simulink model "Model"  (R2024a)
settings: Solver=VariableStepAuto  StartTime=0.0  StopTime=30  RelTol=1e-3
values from neighbouring files (symbols this model uses):
  u_trim = ZStar(10:13)    [Trim_UAV.m]    (also in main.m)
  x_trim = ZStar(1:9)    [Trim_UAV.m]    (also in main.m)
undefined symbols (not defined in the file or in its folder): P, UAV_Morphing_MODEL
libraries: sharedtransform x1
settings Model: Creator=Mustafa Taha  LastModifiedBy=Mustafa Taha

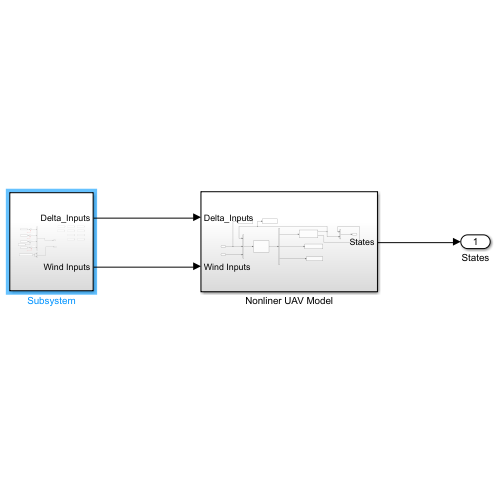
[thumbnail: Simulink's stored preview of the top-level diagram]
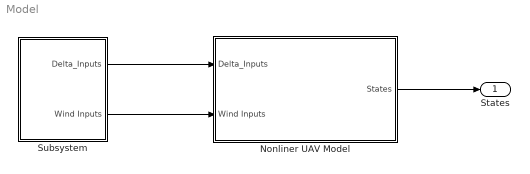
== system Model ==
  Nonliner UAV Model : Subsystem
  Subsystem : Subsystem
  States : Outport
  wires:
  Nonliner UAV Model/1(States) -> States/1
  Subsystem/1(Delta_Inputs) -> Nonliner UAV Model/1(Delta_Inputs)
  Subsystem/2(Wind Inputs) -> Nonliner UAV Model/2(Wind Inputs)

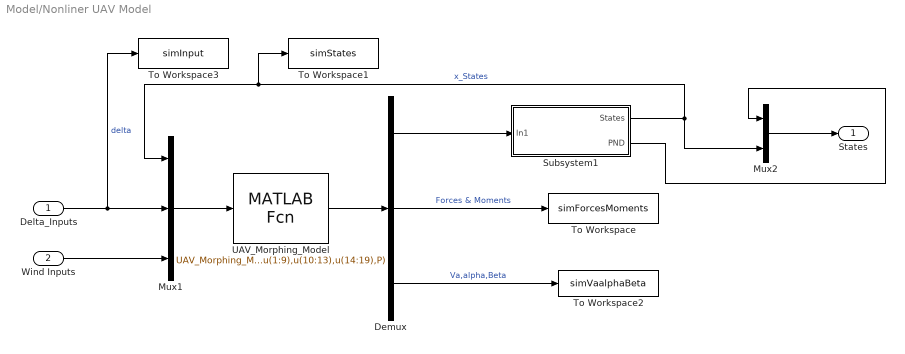
== system Model/Nonliner UAV Model ==
  Delta_Inputs : Inport
  Wind Inputs : Inport  Port=2
  Demux : Demux  Outputs=[9;6;6]
  Mux1 : Mux  Inputs=3
  Mux2 : Mux  Inputs=2
  Subsystem1 : Subsystem
  To Workspace : ToWorkspace  VariableName=simForcesMoments  SaveFormat=Timeseries  SampleTime=-1
  To Workspace1 : ToWorkspace  VariableName=simStates  SaveFormat=Timeseries  SampleTime=-1
  To Workspace2 : ToWorkspace  VariableName=simVaalphaBeta  SaveFormat=Timeseries  SampleTime=-1
  To Workspace3 : ToWorkspace  VariableName=simInput  SaveFormat=Timeseries  SampleTime=-1
  UAV_Morphing_Model : MATLABFcn  MATLABFcn=UAV_Morphing_MODEL(u(1:9),u(10:13),u(14:19),P)  OutputDimensions=21
  States : Outport
  wires:
  Mux1/1 -> UAV_Morphing_Model/1
  Demux/1 -> Subsystem1/1(In1)
  Subsystem1/1(States) -> Mux2/2, To Workspace1/1, Mux1/1  "x_States"
  Wind Inputs/1 -> Mux1/3
  Subsystem1/2(PND) -> Mux2/1
  UAV_Morphing_Model/1 -> Demux/1
  Demux/2 -> To Workspace/1  "Forces & Moments"
  Demux/3 -> To Workspace2/1  "Va,alpha,Beta"
  Mux2/1 -> States/1
  Delta_Inputs/1 -> To Workspace3/1, Mux1/2  "delta"

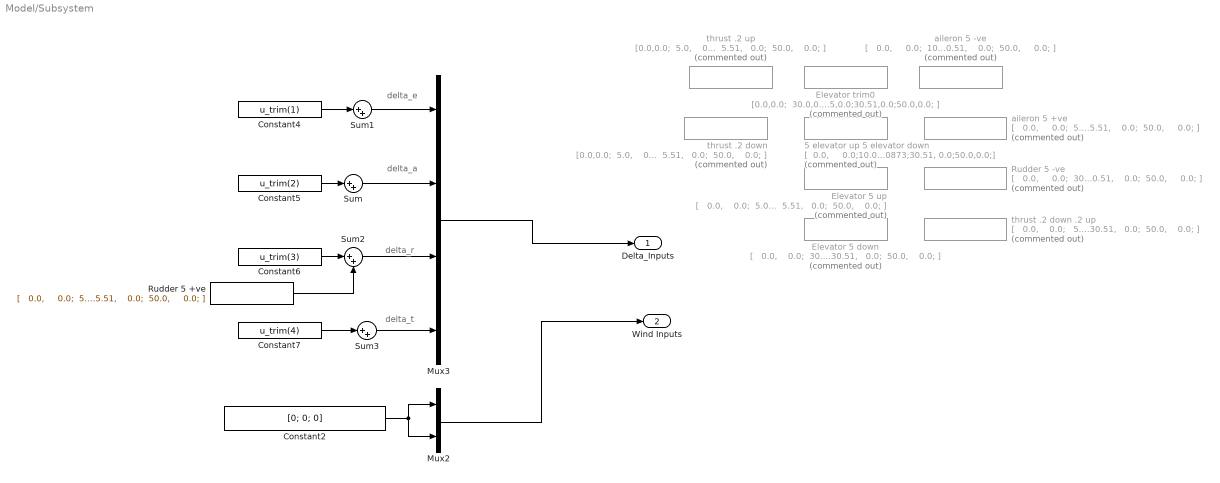
== system Model/Subsystem ==
  note: delta_a
  note: delta_t
  note: delta_e
  note: delta_r
  5 elevator up 5 elevator down : FromWorkspace  Commented=on  VariableName="[  0.0,     0.0;10.0, 0.0;10.01,  -0.0873;10.5,   -0.0873; 10.51,   0.0;30.0,    0.0;30.01,   0.0873;30.5,    0.0873;30.51, 0.0;50.0,0.0;]"
  Constant2 : Constant  Value=[0; 0; 0]
  Constant4 : Constant  Value=u_trim(1)
  Constant5 : Constant  Value=u_trim(2)
  Constant6 : Constant  Value=u_trim(3)
  Constant7 : Constant  Value=u_trim(4)
  Elevator 5 down : FromWorkspace  Commented=on  VariableName=|
      | [
      |   0.0,    0.0;
      |  30.0,    0.0;
      |  30.01,   0.0873;
      |  30.5,    0.0873;
      |  30.51,   0.0;
      |  50.0,    0.0;
      | ]
  Elevator 5 up : FromWorkspace  Commented=on  VariableName=|
      | [
      |   0.0,    0.0;
      |  5.0,    0.0;
      |  5.01,   -0.0873;
      |  5.5,   -0.0873;
      |  5.51,   0.0;
      |  50.0,    0.0;
      | ]
  Elevator trim0 : FromWorkspace  Commented=on  VariableName=|
      | [0.0,0.0;
      |  30.0,0.0;30.01,0.0;30.5,0.0;30.51,0.0;50.0,0.0;
      | ]
  Mux2 : Mux  Inputs=2
  Mux3 : Mux
  Rudder 5 +ve : FromWorkspace  VariableName=|
      | [
      |   0.0,     0.0;
      |  5.0,     0.0;
      |  5.01,   0.0873;
      |  5.5,    0.0873;
      |  5.51,    0.0;
      |  50.0,     0.0;
      | ]
  Rudder 5 -ve : FromWorkspace  Commented=on  VariableName=|
      | [
      |   0.0,     0.0;
      |  30.0,     0.0;
      |  30.01,   -0.0873;
      |  30.5,    -0.0873;
      |  30.51,    0.0;
      |  50.0,     0.0;
      | ]
  Sum{,1..3} (4 alike) : Sum  Inputs=|++
  aileron 5 +ve : FromWorkspace  Commented=on  VariableName=|
      | [
      |   0.0,     0.0;
      |  5.0,     0.0;
      |  5.01,    0.0873;
      |  5.5,     0.0873;
      |  5.51,    0.0;
      |  50.0,     0.0;
      | ]
  aileron 5 -ve : FromWorkspace  Commented=on  VariableName=|
      | [
      |   0.0,     0.0;
      |  10.0,     0.0;
      |  10.01,   -0.0436;
      |  10.5,    -0.0436;
      |  10.51,    0.0;
      |  50.0,     0.0;
      | ]
  thrust .2 down : FromWorkspace  Commented=on  VariableName=|
      | [0.0,0.0;
      |  5.0,    0.0;
      |  5.01,  -0.2;
      |  5.5,   -0.2;
      |  5.51,   0.0;
      |  50.0,    0.0;
      | ]
  thrust .2 down .2 up : FromWorkspace  Commented=on  VariableName=|
      | [
      |   0.0,    0.0;
      |   5.0,    0.0;
      |   5.01,  0.2;
      |   5.5,   0.2;
      |   5.51,   0.0;
      |  30.0,    0.0;
      |  30.01,   -0.2;
      |  30.5,    -0.2;
      |  30.51,   0.0;
      |  50.0,    0.0;
      | ]
  thrust .2 up : FromWorkspace  Commented=on  VariableName=|
      | [0.0,0.0;
      |  5.0,    0.0;
      |  5.01,  0.2;
      |  5.5,   0.2;
      |  5.51,   0.0;
      |  50.0,    0.0;
      | ]
  Delta_Inputs : Outport
  Wind Inputs : Outport  Port=2
  wires:
  Sum2/1 -> Mux3/3
  Constant2/1 -> Mux2/1, Mux2/2
  Constant6/1 -> Sum2/1
  Sum1/1 -> Mux3/1
  Mux2/1 -> Wind Inputs/1
  Constant7/1 -> Sum3/1
  Constant4/1 -> Sum1/1
  Sum/1 -> Mux3/2
  Constant5/1 -> Sum/1
  Mux3/1 -> Delta_Inputs/1
  Sum3/1 -> Mux3/4
  ? -> Sum/2
  ? -> Sum1/2
  ? -> Sum3/2
  Rudder 5 +ve/1 -> Sum2/2

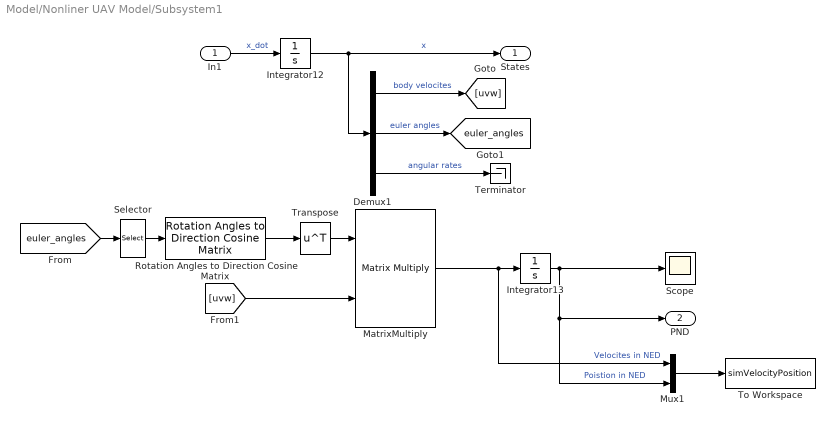
== system Model/Nonliner UAV Model/Subsystem1 ==
  In1 : Inport
  Demux1 : Demux  Outputs=[3,3,3]
  Integrator12 : Integrator  InitialCondition=x_trim
  Integrator13 : Integrator  InitialCondition=[0;0;-100]
  MatrixMultiply : Product  Multiplication=Matrix(*)
  Mux1 : Mux  Inputs=2
  Rotation Angles to Direction Cosine Matrix : sharedtransform/Rotation Angles to Direction Cosine Matrix  rotationOrder=ZYX  aMode=aMode
  Scope : Scope
  Selector : Selector  InputPortWidth=3  IndexOptions=Index vector (dialog)  Indices=[3 2 1]  OutputSizes=1
  Terminator : Terminator
  To Workspace : ToWorkspace  VariableName=simVelocityPosition  SaveFormat=Timeseries  SampleTime=-1
  Transpose : Math  Operator=transpose
  States : Outport
  PND : Outport  Port=2
  tag scope: euler_angles=global
  wires:
  In1/1 -> Integrator12/1  "x_dot"
  Integrator12/1 -> Demux1/1, States/1  "x"
  Integrator13/1 -> PND/1, Mux1/2, Scope/1  "Poistion in NED"
  [euler_angles] -> Selector/1
  Selector/1 -> Rotation Angles to Direction Cosine Matrix/1
  Rotation Angles to Direction Cosine Matrix/1 -> Transpose/1
  [uvw] -> MatrixMultiply/2
  Transpose/1 -> MatrixMultiply/1
  MatrixMultiply/1 -> Mux1/1, Integrator13/1  "Velocites in NED"
  Demux1/1 -> [uvw]  "body velocites"
  Demux1/2 -> [euler_angles]  "euler angles"
  Demux1/3 -> Terminator/1  "angular rates"
  Mux1/1 -> To Workspace/1
